simulink model "roundabout_try1"  (R2016b)
settings: Solver=VariableStepAuto  StartTime=0.0  StopTime=inf  RelTol=1e-3
undefined symbols (not defined in the file): DiscIntNeverNeededParam, vehicle_name
libraries: simulink x7, SCANeR_API x5
settings Model: Creator=z041288  LastModifiedBy=z041288

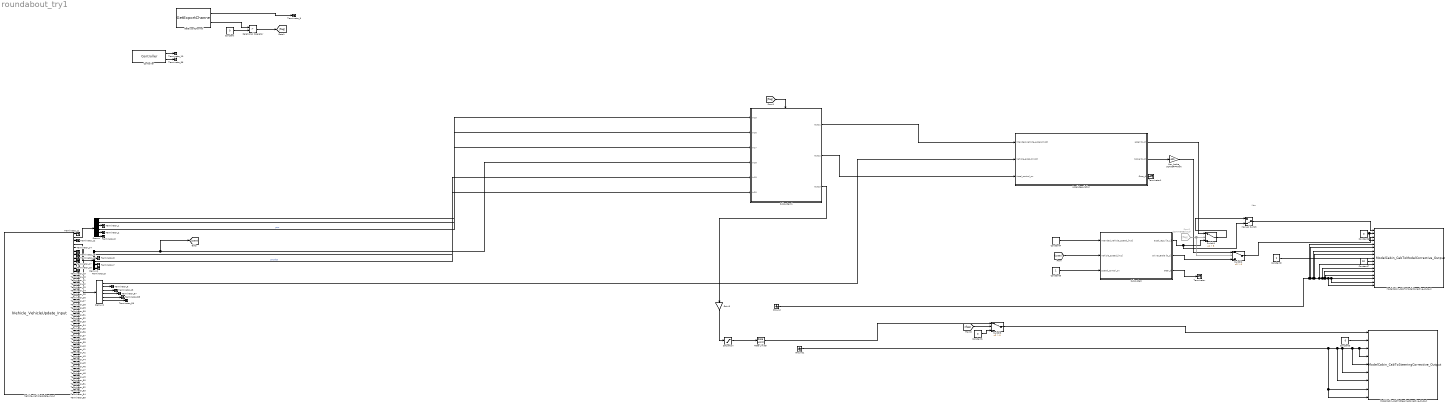
== system roundabout_try1 ==
  note: Man
  Accel_Regulation : Subsystem
  Constant{,1,3,6} (4 alike) : Constant  Value=0
  Constant2 : Constant
  Constant4 : Constant  Value=20*5/18
  Constant5 : Constant
  Constant7 : Constant  Value=10
  Controller : SCANeR_API/Controller  Priority=1  Config='NEWCONFIG_Training'  ProcName='SIMULINK'  Frequency=100  NetworkOutputFrequency=100  TimeOut=3000  IsSynchronized=on
  Demux : Demux  Outputs=6
  Demux1 : Demux  Outputs=6
  Demux2 : Demux  Outputs=6
  From2 : From  Commented=on  GotoTag=flag
  Gain3 : Gain  Gain=1/57
  GetExportChannel : SCANeR_API/GetExportChannel  Priority=0  ExportChannelCategory='debug'  ExportChannelName='SF_debug_001'  VehicleId=-1
  Ground : Ground
  Ground1 : Ground
  IVehicle_VehicleUpdate_Input : SCANeR_API/Network inputs/IVehicle/IVehicle_VehicleUpdate_Input  Priority=2  ev=off  vhlId=0
  Manual Switch : ManualSwitch  CurrentSetting=0
  Max_brake_SCANeR=400N : Gain  Gain=400
  ModelCabin_CabToModelCorrective_Output : SCANeR_API/SHM outputs/ModelCabin/ModelCabin_CabToModelCorrective_Output  Priority=2  shmId=0
  ModelCabin_CabToSteeringCorrective_Output : SCANeR_API/SHM outputs/ModelCabin/ModelCabin_CabToSteeringCorrective_Output  Priority=2  shmId=0
  Rate Limiter : RateLimiter  RisingSlewLimit=10  FallingSlewLimit=-10  SampleTimeMode=inherited
  Relational Operator : RelationalOperator  Operator=>  OutDataTypeStr=boolean  RndMeth=Simplest
  Saturation : Saturate  UpperLimit=10  LowerLimit=-10
  Subsystem : Subsystem
  Subsystem1 : Subsystem
  Switch1 : Switch  Criteria=u2 > Threshold  Threshold=5
  Switch2 : Switch  Criteria=u2 > Threshold
  Switch3 : Switch  Criteria=u2 > Threshold
  Terminator : Terminator
  Terminator1 : Terminator
  Terminator_{1..3,5..59} (58 alike) : Terminator
  wires:
  GetExportChannel/1 -> Terminator_9/1
  GetExportChannel/2 -> Relational Operator/1
  Constant/1 -> Relational Operator/2
  Controller/1 -> Terminator_10/1
  Controller/2 -> Terminator_56/1
  IVehicle_VehicleUpdate_Input/2 -> Demux/1
  IVehicle_VehicleUpdate_Input/4 -> Demux1/1
  Gain3/1 -> Saturation/1
  Ground1/1 -> ModelCabin_CabToSteeringCorrective_Output/8, ModelCabin_CabToSteeringCorrective_Output/9, ModelCabin_CabToSteeringCorrective_Output/4, ModelCabin_CabToSteeringCorrective_Output/3, ModelCabin_CabToSteeringCorrective_Output/5, ModelCabin_CabToSteeringCorrective_Output/6, ModelCabin_CabToSteeringCorrective_Output/7
  Demux/3 -> Terminator_1/1
  Demux/5 -> Terminator_2/1
  Demux/6 -> Terminator_3/1
  Demux1/3 -> Terminator_5/1
  Demux1/5 -> Terminator_7/1
  Demux1/6 -> Terminator_8/1
  IVehicle_VehicleUpdate_Input/1 -> Terminator_11/1
  IVehicle_VehicleUpdate_Input/3 -> Terminator_12/1
  IVehicle_VehicleUpdate_Input/5 -> Demux2/1
  IVehicle_VehicleUpdate_Input/6 -> Terminator_14/1
  IVehicle_VehicleUpdate_Input/7 -> Terminator_15/1
  IVehicle_VehicleUpdate_Input/8 -> Terminator_16/1
  IVehicle_VehicleUpdate_Input/9 -> Terminator_17/1
  IVehicle_VehicleUpdate_Input/10 -> Terminator_18/1
  IVehicle_VehicleUpdate_Input/11 -> Terminator_19/1
  IVehicle_VehicleUpdate_Input/12 -> Terminator_20/1
  IVehicle_VehicleUpdate_Input/13 -> Terminator_21/1
  IVehicle_VehicleUpdate_Input/14 -> Terminator_22/1
  IVehicle_VehicleUpdate_Input/15 -> Terminator_23/1
  IVehicle_VehicleUpdate_Input/16 -> Terminator_24/1
  IVehicle_VehicleUpdate_Input/17 -> Terminator_25/1
  IVehicle_VehicleUpdate_Input/18 -> Terminator_26/1
  IVehicle_VehicleUpdate_Input/19 -> Terminator_27/1
  IVehicle_VehicleUpdate_Input/20 -> Terminator_28/1
  IVehicle_VehicleUpdate_Input/21 -> Terminator_29/1
  IVehicle_VehicleUpdate_Input/22 -> Terminator_30/1
  IVehicle_VehicleUpdate_Input/23 -> Terminator_31/1
  IVehicle_VehicleUpdate_Input/24 -> Terminator_32/1
  IVehicle_VehicleUpdate_Input/25 -> Terminator_33/1
  IVehicle_VehicleUpdate_Input/26 -> Terminator_34/1
  IVehicle_VehicleUpdate_Input/27 -> Terminator_35/1
  IVehicle_VehicleUpdate_Input/28 -> Terminator_36/1
  IVehicle_VehicleUpdate_Input/29 -> Terminator_37/1
  IVehicle_VehicleUpdate_Input/30 -> Terminator_38/1
  IVehicle_VehicleUpdate_Input/31 -> Terminator_39/1
  IVehicle_VehicleUpdate_Input/32 -> Terminator_40/1
  IVehicle_VehicleUpdate_Input/33 -> Terminator_41/1
  IVehicle_VehicleUpdate_Input/34 -> Terminator_42/1
  IVehicle_VehicleUpdate_Input/35 -> Terminator_43/1
  IVehicle_VehicleUpdate_Input/36 -> Terminator_44/1
  IVehicle_VehicleUpdate_Input/37 -> Terminator_45/1
  IVehicle_VehicleUpdate_Input/38 -> Terminator_46/1
  IVehicle_VehicleUpdate_Input/39 -> Terminator_47/1
  IVehicle_VehicleUpdate_Input/40 -> Terminator_48/1
  IVehicle_VehicleUpdate_Input/41 -> Terminator_49/1
  IVehicle_VehicleUpdate_Input/42 -> Terminator_50/1
  IVehicle_VehicleUpdate_Input/43 -> Terminator_51/1
  IVehicle_VehicleUpdate_Input/44 -> Terminator_52/1
  IVehicle_VehicleUpdate_Input/45 -> Terminator_53/1
  IVehicle_VehicleUpdate_Input/46 -> Terminator_54/1
  IVehicle_VehicleUpdate_Input/47 -> Terminator_55/1
  Ground/1 -> ModelCabin_CabToModelCorrective_Output/5, ModelCabin_CabToModelCorrective_Output/6, ModelCabin_CabToModelCorrective_Output/7, ModelCabin_CabToModelCorrective_Output/8, ModelCabin_CabToModelCorrective_Output/11, ModelCabin_CabToModelCorrective_Output/12, ModelCabin_CabToModelCorrective_Output/13, ModelCabin_CabToModelCorrective_Output/14, ModelCabin_CabToModelCorrective_Output/17, ModelCabin_CabToModelCorrective_Output/16, ModelCabin_CabToModelCorrective_Output/15
  Demux1/1 -> Subsystem1/4(In18), [speed]
  Saturation/1 -> Rate Limiter/1
  Demux2/1 -> Accel_Regulation/2(Vehicle_accel_[m/s2])
  Accel_Regulation/2(brake [0_1]) -> Max_brake_SCANeR=400N/1
  Demux2/2 -> Terminator_6/1
  Demux2/3 -> Terminator_13/1
  Demux2/4 -> Terminator_57/1
  Demux2/5 -> Terminator_58/1
  Demux2/6 -> Terminator_59/1
  Constant2/1 -> ModelCabin_CabToModelCorrective_Output/9
  Constant3/1 -> ModelCabin_CabToSteeringCorrective_Output/2
  Constant4/1 -> Subsystem/1(Intended_Vehicle_Speed_[m/s])
  Constant5/1 -> Subsystem/3(Speed_control_on)
  [speed] -> Subsystem/2(Vehicle_Speed_[m/s])
  Accel_Regulation/1(accel [0_1]) -> Switch1/1
  Subsystem/1(accel_regul [0_1]) -> Manual Switch/2, Switch1/3
  Switch1/1 -> Manual Switch/1
  Constant6/1 -> ModelCabin_CabToModelCorrective_Output/4, ModelCabin_CabToModelCorrective_Output/2
  Constant7/1 -> ModelCabin_CabToModelCorrective_Output/10
  Max_brake_SCANeR=400N/1 -> Switch2/1
  Subsystem/2(Driver_Brake [0_1]) -> Switch2/3
  Switch2/1 -> ModelCabin_CabToModelCorrective_Output/3
  Relational Operator/1 -> [flag]
  From2/1 -> Switch1/2, Switch2/2
  Subsystem/3(Gear_d) -> Terminator/1
  Accel_Regulation/3(Gear_d) -> Terminator1/1
  Demux/1 -> Subsystem1/1(In15)
  Demux/2 -> Subsystem1/2(In16)
  Demux/4 -> Subsystem1/3(In17)  "yaw"
  Demux1/2 -> Subsystem1/5(In19)
  Demux1/4 -> Subsystem1/6(In20)  "yawdot"
  Subsystem1/1(Out11) -> Accel_Regulation/1(Intended_Vehicle_accel_[m/s2])
  Subsystem1/2(Out12) -> Accel_Regulation/3(Accel_control_on)
  Subsystem1/3(Out13) -> Gain3/1
  [flag] -> Subsystem1/Enable
  Rate Limiter/1 -> Switch3/1
  Switch3/1 -> ModelCabin_CabToSteeringCorrective_Output/1
  [flag] -> Switch3/2
  Constant1/1 -> Switch3/3
  Manual Switch/1 -> ModelCabin_CabToModelCorrective_Output/1

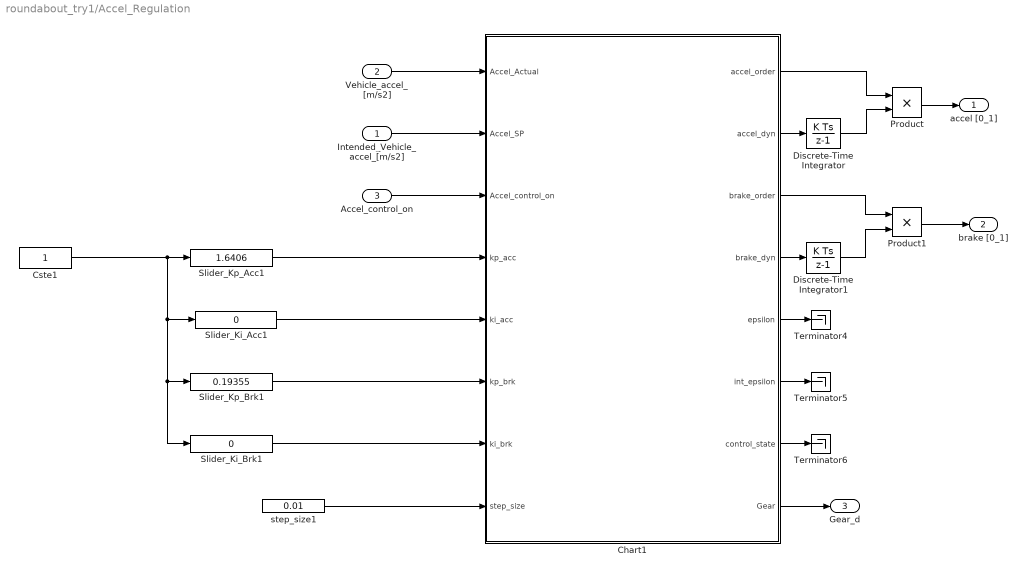
== system roundabout_try1/Accel_Regulation ==
  Intended_Vehicle_accel_[m/s2] : Inport
  Vehicle_accel_[m/s2] : Inport  Port=2
  Accel_control_on : Inport  Port=3
  Chart1 : Stateflow chart  TreatAsAtomicUnit=on  SystemSampleTime=0.01
  Cste1 : Constant  SampleTime=0.01
  Discrete-Time Integrator : DiscreteIntegrator  SampleTime=-1  LimitOutput=on  UpperSaturationLimit=1  LowerSaturationLimit=0  ICPrevOutput=DiscIntNeverNeededParam  ICPrevScaledInput=DiscIntNeverNeededParam
  Discrete-Time Integrator1 : DiscreteIntegrator  SampleTime=-1  LimitOutput=on  UpperSaturationLimit=1  LowerSaturationLimit=0  ICPrevOutput=DiscIntNeverNeededParam  ICPrevScaledInput=DiscIntNeverNeededParam
  Product : Product
  Product1 : Product
  Slider_Ki_Acc1 : simulink/Math Operations/Slider Gain  low=0  gain=0  high=2
  Slider_Ki_Brk1 : simulink/Math Operations/Slider Gain  low=0  gain=0  high=2
  Slider_Kp_Acc1 : simulink/Math Operations/Slider Gain  low=0  gain=1.6406  high=10
  Slider_Kp_Brk1 : simulink/Math Operations/Slider Gain  low=0  gain=0.19355  high=2
  Terminator4 : Terminator
  Terminator5 : Terminator
  Terminator6 : Terminator
  step_size1 : Constant  Value=0.01  SampleTime=0.01
  accel [0_1] : Outport
  brake [0_1] : Outport  Port=2
  Gear_d : Outport  Port=3
  wires:
  Intended_Vehicle_accel_[m/s2]/1 -> Chart1/2(Accel_SP)
  Vehicle_accel_[m/s2]/1 -> Chart1/1(Accel_Actual)
  Accel_control_on/1 -> Chart1/3(Accel_control_on)
  step_size1/1 -> Chart1/8(step_size)
  Chart1/5(epsilon) -> Terminator4/1
  Chart1/6(int_epsilon) -> Terminator5/1
  Slider_Kp_Acc1/1 -> Chart1/4(kp_acc)
  Slider_Ki_Acc1/1 -> Chart1/5(ki_acc)
  Slider_Ki_Brk1/1 -> Chart1/7(ki_brk)
  Slider_Kp_Brk1/1 -> Chart1/6(kp_brk)
  Cste1/1 -> Slider_Ki_Acc1/1, Slider_Kp_Brk1/1, Slider_Ki_Brk1/1, Slider_Kp_Acc1/1
  Chart1/4(brake_dyn) -> Discrete-Time Integrator1/1
  Chart1/2(accel_dyn) -> Discrete-Time Integrator/1
  Chart1/1(accel_order) -> Product/1
  Discrete-Time Integrator/1 -> Product/2
  Product/1 -> accel [0_1]/1
  Chart1/3(brake_order) -> Product1/1
  Discrete-Time Integrator1/1 -> Product1/2
  Product1/1 -> brake [0_1]/1
  Chart1/7(control_state) -> Terminator6/1
  Chart1/8(Gear) -> Gear_d/1

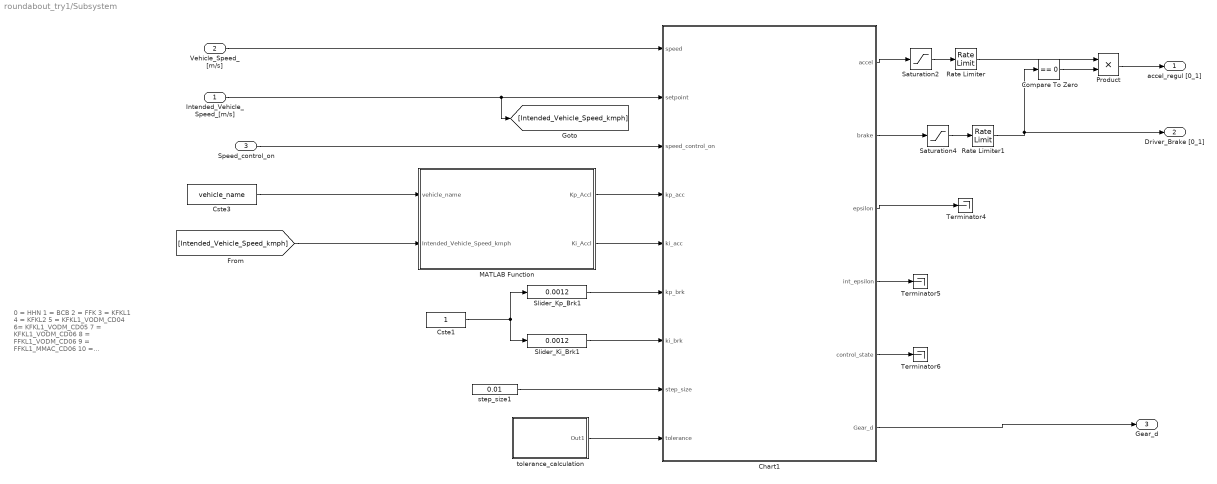
== system roundabout_try1/Subsystem ==
  note: 0 = HHN
      | 1 = BCB
      | 2 = FFK
      | 3 = KFKL1
      | 4 = KFKL2
      | 5 = KFKL1_VODM_CD04
      | 6= KFKL1_VODM_CD05
      | 7 = KFKL1_VODM_CD06
      | 8 = FFKL1_VODM_CD06
      | 9 = FFKL1_MMAC_CD06
      | 10 = FFKL2_MMAC_CD06
      | 11 = KFKL2_MMAC_CD06
      | 12 = XDD_35T_TRS_L2H2
  Intended_Vehicle_Speed_[m/s] : Inport
  Vehicle_Speed_[m/s] : Inport  Port=2
  Speed_control_on : Inport  Port=3
  Chart1 : Stateflow chart  TreatAsAtomicUnit=on  SystemSampleTime=0.01
  Compare To Zero : simulink/Logic and Bit Operations/Compare To Zero  relop===  OutDataTypeStr=boolean
  Cste1 : Constant  SampleTime=0.01
  Cste3 : Constant  Value=vehicle_name  SampleTime=0.01
  MATLAB Function : MATLAB Function  TreatAsAtomicUnit=on
  Product : Product
  Rate Limiter : RateLimiter  RisingSlewLimit=0.5  SampleTimeMode=inherited
  Rate Limiter1 : RateLimiter  RisingSlewLimit=0.2  SampleTimeMode=inherited
  Saturation2 : Saturate  UpperLimit=1  LowerLimit=0  SampleTime=0.01
  Saturation4 : Saturate  UpperLimit=1  LowerLimit=0  SampleTime=0.01
  Slider_Ki_Brk1 : simulink/Math Operations/Slider Gain  low=0  gain=0.0012  high=2
  Slider_Kp_Brk1 : simulink/Math Operations/Slider Gain  low=0  gain=0.0012  high=1
  Terminator4 : Terminator
  Terminator5 : Terminator
  Terminator6 : Terminator
  step_size1 : Constant  Value=0.01  SampleTime=0.01
  tolerance_calculation : Subsystem
  accel_regul [0_1] : Outport
  Driver_Brake [0_1] : Outport  Port=2
  Gear_d : Outport  Port=3
  wires:
  Cste1/1 -> Slider_Kp_Brk1/1, Slider_Ki_Brk1/1
  Slider_Kp_Brk1/1 -> Chart1/6(kp_brk)
  Slider_Ki_Brk1/1 -> Chart1/7(ki_brk)
  MATLAB Function/2(Ki_Accl) -> Chart1/5(ki_acc)
  MATLAB Function/1(Kp_Accl) -> Chart1/4(kp_acc)
  Chart1/5(control_state) -> Terminator6/1
  Chart1/4(int_epsilon) -> Terminator5/1
  Chart1/3(epsilon) -> Terminator4/1
  Chart1/2(brake) -> Saturation4/1
  step_size1/1 -> Chart1/8(step_size)
  Saturation4/1 -> Rate Limiter1/1
  Vehicle_Speed_[m/s]/1 -> Chart1/1(speed)
  Intended_Vehicle_Speed_[m/s]/1 -> [Intended_Vehicle_Speed_kmph], Chart1/2(setpoint)
  Saturation2/1 -> Rate Limiter/1
  Rate Limiter/1 -> Product/1
  Product/1 -> accel_regul [0_1]/1
  Rate Limiter1/1 -> Compare To Zero/1, Driver_Brake [0_1]/1
  Chart1/6(Gear_d) -> Gear_d/1
  Speed_control_on/1 -> Chart1/3(speed_control_on)
  Cste3/1 -> MATLAB Function/1(vehicle_name)
  [Intended_Vehicle_Speed_kmph] -> MATLAB Function/2(Intended_Vehicle_Speed_kmph)
  Compare To Zero/1 -> Product/2
  Chart1/1(accel) -> Saturation2/1
  tolerance_calculation/1(Out1) -> Chart1/9(tolerance)

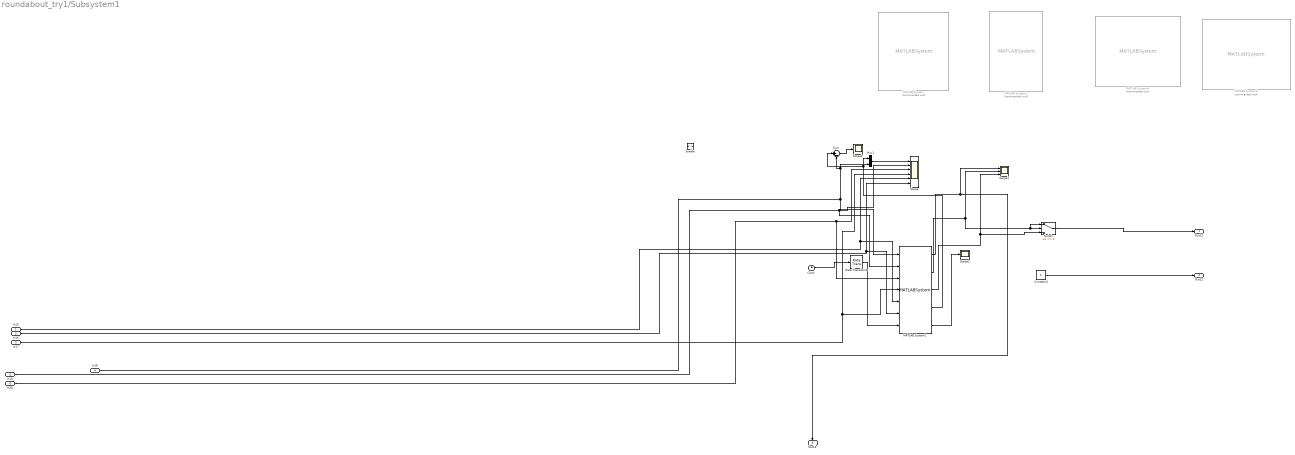
== system roundabout_try1/Subsystem1 ==
  In15 : Inport
  In16 : Inport  Port=2
  In17 : Inport  Port=3
  In18 : Inport  Port=4
  In19 : Inport  Port=5
  In20 : Inport  Port=6
  Enable : EnablePort
  Clock : Clock
  Constant1 : Constant
  MATLAB System : MATLABSystem  Commented=on  System=casadi_block_MPCtry_1  SimulateUsing=Interpreted execution
      mask Type: casadi_block_MPCtry_1
      mask Display:
      | disp('casadi_block_MPCtry_1');
      | port_label('input',1,'xd_in');
      | port_label('input',2,'yd_in');
      | port_label('input',3,'yawd_in');
      | port_label('input',4,'yaw_in');
      | port_label('input',5,'x_in');
      | port_label('input',6,'y_in');
      | port_label('input',7,'t');
      | port_label('output',1,'delta_out');
      | port_label('output',2,'acc_out');
      | port_label('output',3,'break_out');
      | port_label('output',4,'vref');
      | port_label('output',5,'err');
  MATLAB System1 : MATLABSystem  System=casadi_block_MPCtry_3  SimulateUsing=Interpreted execution
      mask Type: casadi_block_MPCtry_3
      mask Display:
      | disp('casadi_block_MPCtry_3');
      | port_label('input',1,'xd_in');
      | port_label('input',2,'yd_in');
      | port_label('input',3,'yawd_in');
      | port_label('input',4,'yaw_in');
      | port_label('input',5,'x_in');
      | port_label('input',6,'y_in');
      | port_label('input',7,'t');
      | port_label('output',1,'delta_out');
      | port_label('output',2,'acc_out');
      | port_label('output',3,'break_out');
      | port_label('output',4,'vref');
      | port_label('output',5,'err');
  MATLAB System2 : MATLABSystem  Commented=on  System=casadi_block_MPC_LSS  SimulateUsing=Interpreted execution
      mask Type: casadi_block_MPC_LSS
      mask Display:
      | disp('casadi_block_MPC_LSS');
      | port_label('input',1,'xd_in');
      | port_label('input',2,'yd_in');
      | port_label('input',3,'yawd_in');
      | port_label('input',4,'yaw_in');
      | port_label('input',5,'x_in');
      | port_label('input',6,'y_in');
      | port_label('input',7,'t');
      | port_label('output',1,'delta_out');
      | port_label('output',2,'acc_out');
      | port_label('output',3,'break_out');
      | port_label('output',4,'vref');
      | port_label('output',5,'err');
  MATLAB System3 : MATLABSystem  Commented=on  System=casadi_block_MPC_left_turn  SimulateUsing=Interpreted execution
      mask Type: casadi_block_MPC_left_turn
      mask Display:
      | disp('casadi_block_MPC_left_turn');
      | port_label('input',1,'xd_in');
      | port_label('input',2,'yd_in');
      | port_label('input',3,'yawd_in');
      | port_label('input',4,'yaw_in');
      | port_label('input',5,'x_in');
      | port_label('input',6,'y_in');
      | port_label('input',7,'t');
      | port_label('output',1,'delta_out');
      | port_label('output',2,'acc_out');
      | port_label('output',3,'break_out');
      | port_label('output',4,'vref');
      | port_label('output',5,'err');
  MATLAB System4 : MATLABSystem  Commented=on  System=casadi_block_MPC_left_turn_2  SimulateUsing=Interpreted execution
      mask Type: casadi_block_MPC_left_turn_2
      mask Display:
      | disp('casadi_block_MPC_left_turn_2');
      | port_label('input',1,'xd_in');
      | port_label('input',2,'yd_in');
      | port_label('input',3,'yawd_in');
      | port_label('input',4,'yaw_in');
      | port_label('input',5,'x_in');
      | port_label('input',6,'y_in');
      | port_label('input',7,'t');
      | port_label('output',1,'delta_out');
      | port_label('output',2,'acc_out');
      | port_label('output',3,'break_out');
      | port_label('output',4,'vref');
      | port_label('output',5,'err');
  Mux1 : Mux  Inputs=2
  Rate Transition2 : RateTransition  OutPortSampleTime=0.02
  Scope : Scope  NumInputPorts=6
  Scope1 : Scope  NumInputPorts=3
  Scope2 : Scope
  Scope3 : Scope
  Sum : Sum  Inputs=|+-
  Switch : Switch
  Out11 : Outport
  Out12 : Outport  Port=2
  Out13 : Outport  Port=3
  wires:
  In18/1 -> MATLAB System1/1, Sum/2, Mux1/2
  MATLAB System1/1 -> Out13/1, Scope1/1
  In15/1 -> MATLAB System1/5, Scope/5
  In16/1 -> MATLAB System1/6, Scope/6
  In20/1 -> MATLAB System1/3, Scope/3
  In19/1 -> MATLAB System1/2, Scope/2
  MATLAB System1/5 -> Scope2/1
  Rate Transition2/1 -> MATLAB System1/7
  Mux1/1 -> Scope/1
  MATLAB System1/2 -> Switch/1, Switch/2, Scope1/2
  Clock/1 -> Rate Transition2/1
  MATLAB System1/4 -> Sum/1, Mux1/1
  In17/1 -> MATLAB System1/4, Scope/4
  Switch/1 -> Out11/1
  MATLAB System1/3 -> Switch/3, Scope1/3
  Sum/1 -> Scope3/1
  Constant1/1 -> Out12/1

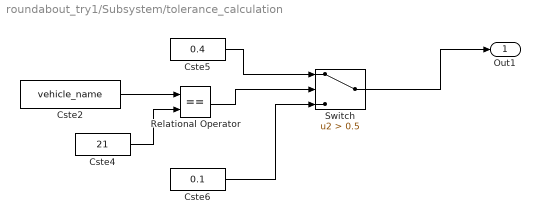
== system roundabout_try1/Subsystem/tolerance_calculation ==
  Cste2 : Constant  Value=vehicle_name  SampleTime=0.01
  Cste4 : Constant  Value=21  SampleTime=0.01
  Cste5 : Constant  Value=0.4  SampleTime=0.01
  Cste6 : Constant  Value=0.1  SampleTime=0.01
  Relational Operator : RelationalOperator  Operator===  OutDataTypeStr=boolean  RndMeth=Simplest
  Switch : Switch  Criteria=u2 > Threshold  Threshold=0.5
  Out1 : Outport
  wires:
  Switch/1 -> Out1/1
  Cste6/1 -> Switch/3
  Cste5/1 -> Switch/1
  Cste2/1 -> Relational Operator/1
  Cste4/1 -> Relational Operator/2
  Relational Operator/1 -> Switch/2

== stateflow chart roundabout_try1/Accel_Regulation/Chart1 ==
  state Accel_Control/
    state Control_Off/
      accel_order= 0;
      brake_order= 0;
      accel_dyn= 0;
      brake_dyn= 0;
      int_epsilon = 0;
      Gear=10;
    state Controller/
      limit_accel = 1/kp_acc;
      limit_brake = 1/kp_brk;
      state Acceleration_regulation/
        state accel/
          control_state = 2;
          accel_order=1;
          brake_order= 0;
          accel_dyn=  kp_acc*epsilon + ki_acc*int_epsilon;
          brake_dyn= 0;
          Gear=10;
        (junction 59) -> accel [order 1] : [abs(epsilon) < limit_accel & control_state == 2]
            | {int_epsilon = int_epsilon + step_size*epsilon;}
        (junction 59) -> accel [order 2] : {int_epsilon = 0;}
      state Brake_regulation/
        state brake/
          control_state = 1;
          accel_order=0;
          brake_order=1;
          accel_dyn= 0;
          brake_dyn=  kp_brk*epsilon + ki_brk*int_epsilon;
          Gear=10;
        (junction 101) -> brake [order 1] : [abs(epsilon) < limit_brake & control_state == 1]
            | {int_epsilon = int_epsilon + step_size*epsilon;}
        (junction 101) -> brake [order 2] : {int_epsilon = 0;}
      accel -> (junction 56)
      brake -> (junction 56)
      (junction 56) -> (junction 59) [order 1] : [Accel_SP >= 0]
          | {epsilon =Accel_SP-Accel_Actual;}
      (junction 56) -> (junction 101) [order 2] : {epsilon =Accel_Actual-Accel_SP;}
    (default) -> (junction 55)
    (junction 55) -> Control_Off [order 1] : [Accel_control_on == 0]
    Control_Off -> (junction 55)
    Controller -> (junction 55) : [Accel_control_on == 0]
    (junction 55) -> (junction 56) [order 2] : {control_state = 0;}
  data: Accel_Actual input double; Accel_SP input double; Accel_control_on input double; accel_order output double; accel_dyn output double; brake_order output double; brake_dyn output double; kp_acc input double; ki_acc input double; kp_brk input double; ki_brk input double; step_size input double; limit_accel local double; limit_brake local double; epsilon output double; int_epsilon output double; control_state output double; Gear output double

== stateflow chart roundabout_try1/Subsystem/Chart1 ==
  state Speed_Control/
    state Control_Off/
      accel = 0;
      brake = 0;
      int_epsilon = 0;
      Gear=3;
    state Controller/
      limit_accel = 1/kp_acc;
      limit_brake = 1/kp_brk;
      state normal_regulation/
        state normal_accel/
          control_state = 2;
          accel = -kp_acc*epsilon - ki_acc*int_epsilon;
          brake = 0;
          Gear_d = Gear;
        state normal_brake/
          control_state = 1;
          brake = kp_brk*epsilon + ki_brk*int_epsilon;
          accel = 0;
          Gear_d = Gear;
        (junction 58) -> (junction 59) [order 1] : [epsilon <= tolerance]
        (junction 58) -> (junction 57) [order 2]
        (junction 59) -> Speed_Control.Controller.normal_regulation.normal_accel [order 1] : [abs(epsilon) < limit_accel & control_state == 2]
            | {int_epsilon = int_epsilon + step_size*epsilon;}
        (junction 59) -> Speed_Control.Controller.normal_regulation.normal_accel [order 2] : {int_epsilon = 0;}
        (junction 57) -> Speed_Control.Controller.normal_regulation.normal_brake [order 1] : [abs(epsilon) < limit_brake & control_state == 1]
            | {int_epsilon = int_epsilon + step_size*epsilon;}
        (junction 57) -> Speed_Control.Controller.normal_regulation.normal_brake [order 2] : {int_epsilon = 0;}
        Speed_Control.Controller.normal_regulation.normal_brake -> (junction 69)
        Speed_Control.Controller.normal_regulation.normal_accel -> (junction 69)
      state reverse_regulation1/
        state normal_accel/
          control_state = 2;
          accel = -kp_acc*epsilon - ki_acc*int_epsilon;
          brake = 0;
          Gear_d = Gear;
        state normal_brake/
          control_state = 1;
          brake = kp_brk*epsilon + ki_brk*int_epsilon;
          accel = 0;
          Gear_d = Gear;
        (junction 123) -> (junction 124) [order 1] : [epsilon <=-0.1]
        (junction 123) -> (junction 125) [order 2]
        (junction 124) -> Speed_Control.Controller.reverse_regulation1.normal_accel [order 1] : [abs(epsilon) < limit_accel & control_state == 2]
            | {int_epsilon = int_epsilon + step_size*epsilon;}
        (junction 124) -> Speed_Control.Controller.reverse_regulation1.normal_accel [order 2] : {int_epsilon = 0;}
        (junction 125) -> Speed_Control.Controller.reverse_regulation1.normal_brake [order 1] : [abs(epsilon) < limit_brake & control_state == 1]
            | {int_epsilon = int_epsilon + step_size*epsilon;}
        (junction 125) -> Speed_Control.Controller.reverse_regulation1.normal_brake [order 2] : {int_epsilon = 0;}
        Speed_Control.Controller.reverse_regulation1.normal_brake -> (junction 126)
        Speed_Control.Controller.reverse_regulation1.normal_accel -> (junction 126)
      (junction 56) -> (junction 99) [order 1] : [setpoint< 0]
          | {epsilon =- speed+setpoint;}
      (junction 56) -> (junction 62) [order 2] : {epsilon = speed-setpoint;}
      (junction 62) -> (junction 58) : {Gear =10;}
      (junction 69) -> (junction 56)
      (junction 126) -> (junction 56)
      (junction 99) -> (junction 123) : {Gear =2;}
    (default) -> (junction 55)
    (junction 55) -> Control_Off [order 1] : [speed_control_on == 0]
    Control_Off -> (junction 55)
    Controller -> (junction 55) : [speed_control_on == 0]
    (junction 55) -> (junction 56) [order 2] : {control_state = 0;}
  data: speed input double; setpoint input double; speed_control_on input double; accel output double; brake output double; kp_acc input double; ki_acc input double; kp_brk input double; ki_brk input double; step_size input double; limit_accel local double; limit_brake local double; epsilon output double; int_epsilon output double; control_state output double; Gear_d output double; Gear local double; tolerance input double

== matlab function roundabout_try1/Subsystem/MATLAB Function ==
  data: vehicle_name input; Kp_Accl output; Ki_Accl output; Intended_Vehicle_Speed_kmph input
function [Kp_Accl, Ki_Accl]= fcn(vehicle_name,Intended_Vehicle_Speed_kmph)
% This function calculates the Kp_Accl and Ki_Accl
% Following are the vehicle models to be used for simulation
% Vehicle_name:
% 0 = HHN
% 1 = BCB
% 2 = FFK
% 3 = KFKL1
% 4 = KFKL2
% 5 = KFKL1_VODM_CD04
% 6= KFKL1_VODM_CD05
% 7 = KFKL1_VODM_CD06
% 8 = FFKL1_VODM_CD06
% 9 = FFKL1_MMAC_CD06
% 10 = FFKL2_MMAC_CD06
% 11 = KFKL2_MMAC_CD06
% 12 = XDD

if (vehicle_name == 0)
    Kp_Accl = 0.3;
    Ki_Accl = 0.05;
elseif (vehicle_name == 1)
    Kp_Accl = 0.3;
    Ki_Accl = 0.05;
elseif (vehicle_name == 2)
    Kp_Accl = 0.1;
    Ki_Accl = 0.02;
elseif (vehicle_name == 3)
    Kp_Accl = 0.3;
    Ki_Accl = 0.02;
elseif (vehicle_name == 4)
    Kp_Accl = 0.3;
    Ki_Accl = 0.02;
elseif (vehicle_name == 5)
    Kp_Accl = 0.3;
    Ki_Accl = 0.02;
elseif (vehicle_name == 6)
    Kp_Accl = 0.3;
    Ki_Accl = 0.02;
elseif (vehicle_name == 7)
    Kp_Accl = 0.3;
    Ki_Accl = 0.02;
elseif (vehicle_name == 8)
    Kp_Accl = 0.3;
    Ki_Accl = 0.02;
elseif (vehicle_name == 9)
    Kp_Accl = 0.3;
    Ki_Accl = 0.02;
elseif (vehicle_name == 10)
    Kp_Accl = 0.3;
    Ki_Accl = 0.02;
elseif (vehicle_name == 11)
    Kp_Accl = 0.3;
    Ki_Accl = 0.02;
elseif (vehicle_name == 17)% HCB 60kwh
    if Intended_Vehicle_Speed_kmph >= 60
        Kp_Accl = 0.3; %0.1
        Ki_Accl = 0.05;%0.01
    else
        Kp_Accl = 0.1; %0.1
        Ki_Accl = 0.01;%0.01
    end
elseif (vehicle_name == 13) || (vehicle_name == 15) % BCB
    Kp_Accl =0.3;
    Ki_Accl = 0.05;
elseif (vehicle_name == 18) || (vehicle_name == 14) || (vehicle_name == 12)% XDD vehicle
    Kp_Accl = 0.3;
    Ki_Accl = 0.05;
elseif (vehicle_name == 19)% BCB 40kwh Correl
    if Intended_Vehicle_Speed_kmph >= 50
        Kp_Accl = 1;
        Ki_Accl = 0.1;
    else
        Kp_Accl = 0.1; %0.1
        Ki_Accl = 0.01;%0.01
    end
elseif (vehicle_name == 16) % HHN Correl
    if Intended_Vehicle_Speed_kmph >= 15
        Kp_Accl = 0.3;
        Ki_Accl = 0.05;
    elseif Intended_Vehicle_Speed_kmph < 7
        Kp_Accl = 0.3;
        Ki_Accl = 0.05;
    else
        Kp_Accl = 0.009;
        Ki_Accl = 0.00032;
    end
elseif (vehicle_name == 20) % Echo
    Kp_Accl = 0.3;
    Ki_Accl = 0.05;
elseif (vehicle_name == 21) % Torque Management
    Kp_Accl = 0.0012;
    Ki_Accl = 0.0012;
else  % Other vehicles
    if Intended_Vehicle_Speed_kmph >= 15
        Kp_Accl = 0.3;
        Ki_Accl = 0.05;
    else
        Kp_Accl = 0.009;
        Ki_Accl = 0.00032;
    end
end
